simulink subsystem "p5"  (R2020b)
settings: Solver=VariableStepAuto  StartTime=0.0  StopTime=10.0  RelTol=1e-3
settings Model: Creator=nevinliang  LastModifiedBy=nevinliang

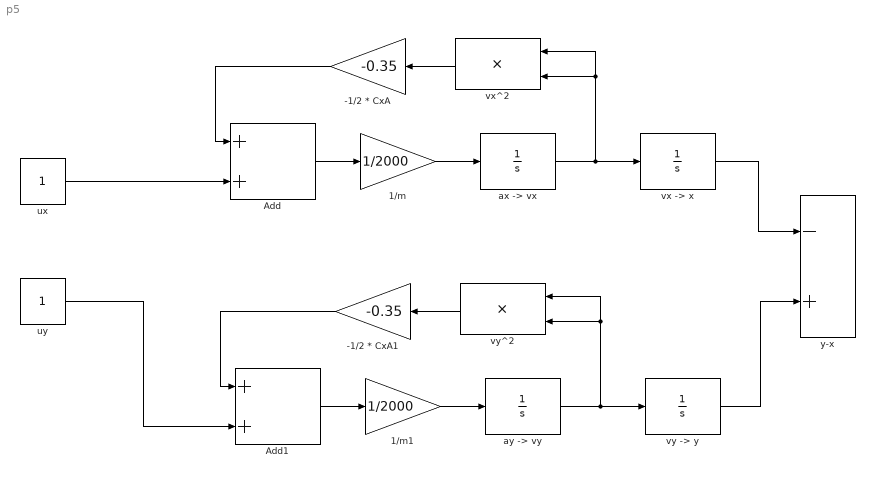
== system p5 ==
  -1/2 * CxA : Gain  Gain=-0.35
  -1/2 * CxA1 : Gain  Gain=-0.35
  1/m : Gain  Gain=1/2000
  1/m1 : Gain  Gain=1/2000
  Add : Sum
  Add1 : Sum
  "ax -> vx" : TransferFcn  Denominator=[1 0]
  "ay -> vy" : TransferFcn  Denominator=[1 0]
  ux : Constant
  uy : Constant
  "vx -> x" : TransferFcn  Denominator=[1 0]
  vx^2 : Product
  "vy -> y" : TransferFcn  Denominator=[1 0]
  vy^2 : Product
  y-x : Sum  Inputs=-+
  wires:
  vx^2/1 -> -1/2 * CxA/1
  "ax -> vx"/1 -> vx^2/1, vx^2/2, "vx -> x"/1
  1/m/1 -> "ax -> vx"/1
  -1/2 * CxA/1 -> Add/1
  Add/1 -> 1/m/1
  Add1/1 -> 1/m1/1
  -1/2 * CxA1/1 -> Add1/1
  uy/1 -> Add1/2
  1/m1/1 -> "ay -> vy"/1
  "vx -> x"/1 -> y-x/1
  "ay -> vy"/1 -> vy^2/1, vy^2/2, "vy -> y"/1
  vy^2/1 -> -1/2 * CxA1/1
  "vy -> y"/1 -> y-x/2
  ux/1 -> Add/2
